simulink model "rocky"  (R2022a)
settings: Solver=VariableStepAuto  StartTime=0.0  StopTime=10.0  RelTol=1e-3
settings Model: Creator=cpark1  LastModifiedBy=cpark1

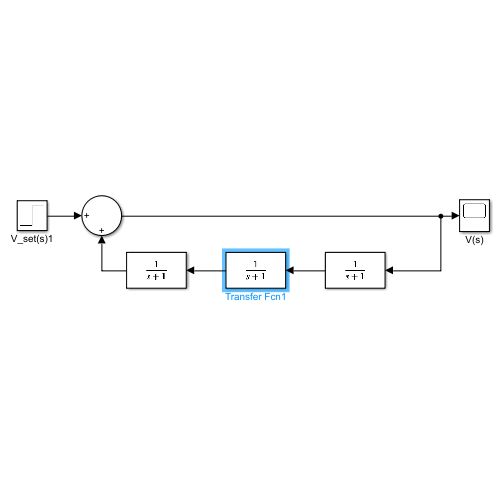
[thumbnail: Simulink's stored preview of the top-level diagram]
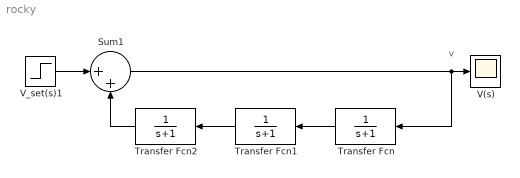
== system rocky ==
  note: v
  Sum1 : Sum  Inputs=|++
  Transfer Fcn : TransferFcn  Denominator=[1 1]
  Transfer Fcn1 : TransferFcn  Denominator=[1 1]
  Transfer Fcn2 : TransferFcn  Denominator=[1 1]
  V(s) : Scope
  V_set(s)1 : Step  Time=0  After=20  SampleTime=0
  wires:
  V_set(s)1/1 -> Sum1/1
  Sum1/1 -> V(s)/1, Transfer Fcn/1
  Transfer Fcn/1 -> Transfer Fcn1/1
  Transfer Fcn1/1 -> Transfer Fcn2/1
  Transfer Fcn2/1 -> Sum1/2
